simulink model "sampleModel298"  (R2021b)
settings: Solver=VariableStepAuto  StartTime=0.0  StopTime=10.0  RelTol=1e-3
libraries: simulink x11, slpidlib x2
settings Model: Creator=user  LastModifiedBy=user

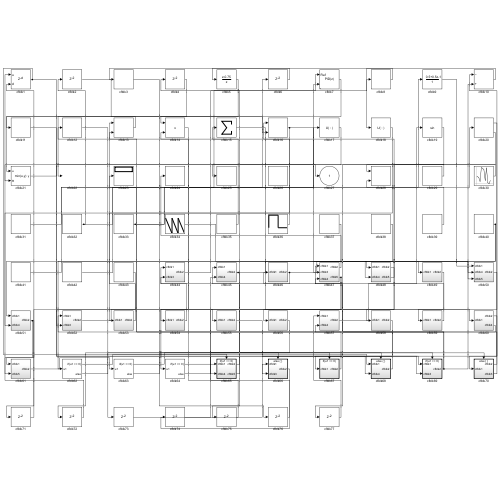
[thumbnail: Simulink's stored preview of the top-level diagram]
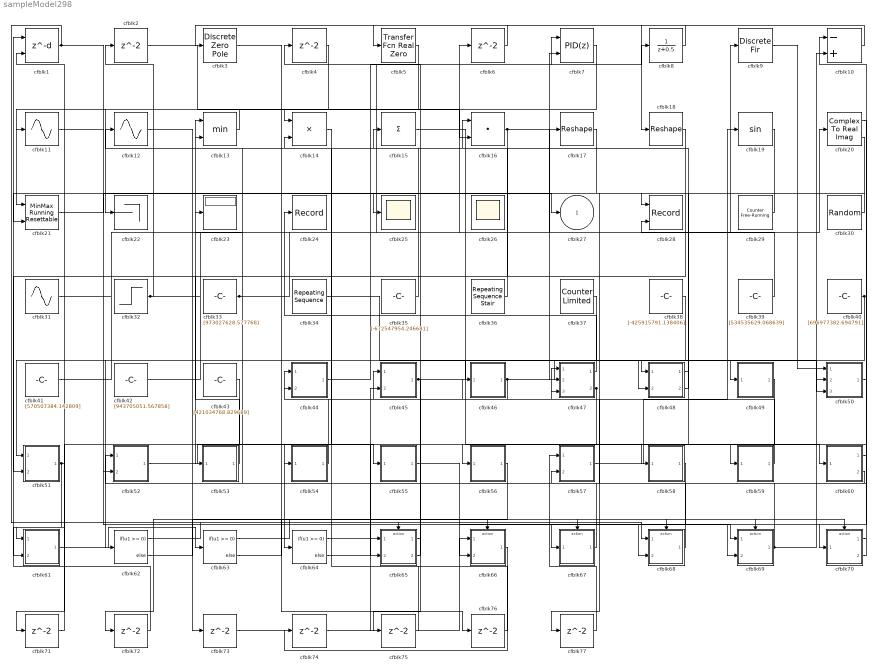
== system sampleModel298 ==
  cfblk1 : Delay  DelayLengthSource=Input port  SampleTime=1
      settings: InputPortMap=u0,p1
  cfblk10 : Sum  Inputs=-+
  cfblk11 : Sin  TimeSource=Use external signal  SampleTime=0
  cfblk12 : Sin  TimeSource=Use external signal  SampleTime=0
  cfblk13 : MinMax  Inputs=2
  cfblk14 : Product
  cfblk15 : Sum  Inputs=+
  cfblk16 : DotProduct  InputSameDT=on  OutDataTypeStr=Inherit: Inherit via internal rule
  cfblk17 : Reshape
  cfblk18 : Reshape
  cfblk19 : Trigonometry
  cfblk{2,4,6,71..77} (10 alike) : Delay  SampleTime=1
  cfblk20 : ComplexToRealImag
  cfblk21 : simulink/Math Operations/MinMax Running Resettable  Function=min  vinit=0.0
  cfblk22 : Terminator
  cfblk23 : Display
  cfblk24 : Record  FileSettingsInternal="{\"entries\":[{\"content\":{\"excelSettings\":{\"content\":{},\"type\":\"Streamout.ExcelSettings\"}},\"type\":\"Streamout.FileSettingStorage\",\"uuid\":\"f8e03bbd-3925-4cbe-a2d8-1c15d8116227\"}],\"packageUris\":[\"http://schema.mathworks.com/mf0/streamout_blocks/R2020a\"],\"version\":\"1.0\"}"  SignalsInternal="{\"entries\":[{\"content\":{\"signals\":[{\"content\":{\"blockPath\":[\"sampleModel298/cfblk24\"],\"channel\":[],\"dimensions\":[1],\"domain\":\"sampleModel298/cfblk24\",\"lineColor\":\"#a2142f\",\"plots\":[1],\"port\":1,\"sid\":[\"\"],\"signalID\":12860,\"signalName\":\"cfblk47:1\"},\"type\":\"RecordBlkView.Signal\",\"uuid\":\"11e5b281-7313-45d0-8552-5ee48f4d8115\"}]},\"type\":\"RecordBlkView.InputSignals\",\"uuid\":\"8eee72e8-d15a-4497-b3c0-09b01b3c1e58\"}],\"packageUris\":[\"http://schema.mathworks.com/mf0/streamout_blocks/R2020a\"],\"version\":\"1.0\"}"  VisualizationBindings="{\"sparklinesplugin\":{\"info\":[{\"bindingParametersList\":[],\"subplotID\":1}]}}"
  cfblk25 : Scope
  cfblk26 : Scope
      settings: Floating=on
  cfblk28 : Record  FileSettingsInternal="{\"entries\":[{\"content\":{\"excelSettings\":{\"content\":{},\"type\":\"Streamout.ExcelSettings\"}},\"type\":\"Streamout.FileSettingStorage\",\"uuid\":\"aa3ee1ba-3106-412b-81ca-2127dd02a330\"}],\"packageUris\":[\"http://schema.mathworks.com/mf0/streamout_blocks/R2020a\"],\"version\":\"1.0\"}"  Layout=[1 1]  SignalsInternal="{\"entries\":[{\"content\":{\"signals\":[{\"content\":{\"blockPath\":[\"sampleModel298/cfblk28\"],\"channel\":[],\"dimensions\":[1],\"domain\":\"sampleModel298/cfblk28\",\"lineColor\":\"#a2142f\",\"plots\":[1],\"port\":1,\"sid\":[\"\"],\"signalID\":12864,\"signalName\":\"cfblk30\"},\"type\":\"RecordBlkView.Signal\",\"uuid\":\"5ab1b331-6bbc-4e8d-9462-f5e53011d17e\"},{\"content\":{\"blockPath\":[\"sampleModel298/cfblk28\"],\"channel\":[],\"dimensions\":[1],\"domain\":\"sampleModel298/cfblk28\",\"lineColor\":\"#139fff\",\"plots\":[1],\"port\":2,\"sid\":[\"\"],\"signalID\":12868,\"signalName\":\"cfblk39\"},\"type\":\"RecordBlkView.Signal\",\"uuid\":\"ca5edff8-c0fa-4e9c-811a-b661a9ca84b8\"}]},\"type\":\"RecordBlkView.InputSignals\",\"uuid\":\"61fdf1d2-9825-4d1b-a59d-4a14db1b4992\"}],\"packageUris\":[\"http://schema.mathworks.com/mf0/streamout_blocks/R2020a\"],\"version\":\"1.0\"}"  VisualizationBindings="{\"xyplotplugin\":{\"info\":[{\"series\":[{\"bindingParametersList\":[{\"parameter\":\"X-Axis\",\"signalID\":12864,\"signalName\":\"cfblk30\"},{\"parameter\":\"Y-Axis\",\"signalID\":12868,\"signalName\":\"cfblk39\"}],\"seriesID\":55334}],\"subplotID\":1}]}}"  CompatibilityTag=XY
  cfblk29 : simulink/Sources/Counter Free-Running  NumBits=[26.000000]  tsamp=-1
  cfblk3 : DiscreteZeroPole  Poles=[0 0.5]  Gain=1
  cfblk30 : RandomNumber  Mean=[-77149.220000]  Variance=[41680.275805]  Seed=[340606104.000000]  SampleTime=0.1
  cfblk31 : Sin  Amplitude=[967904790.389444]  Bias=[-694401713.764800]  SampleTime=0
  cfblk32 : Step  Time=[28.000000]  Before=[-871235636.671696]  After=[850693744.630323]  SampleTime=0
  cfblk33 : Constant  Value=[973027628.577768]  SampleTime=1
  cfblk34 : simulink/Sources/Repeating Sequence  rep_seq_t=[0 2]  rep_seq_y=[-129325403.939381, -689316704.616454]
  cfblk35 : Constant  Value=[-672547954.246681]  SampleTime=1
  cfblk36 : simulink/Sources/Repeating Sequence Stair  OutValues=[-374108966.270243, -413875160.469731]  tsamp=-1  OutMin=[]  OutMax=[]  OutDataTypeStr=double  OutputDataTypeScalingMode=double  OutDataType=fixdt(0,8)  ConRadixGroup=Best Precision: Vector-wise  OutScaling=2^-12
  cfblk37 : simulink/Sources/Counter Limited  uplimit=[389.000000]  tsamp=-1
  cfblk38 : Constant  Value=[-425915791.138406]  SampleTime=1
  cfblk39 : Constant  Value=[534535629.068639]  SampleTime=1
  cfblk40 : Constant  Value=[696977382.694791]  SampleTime=1
  cfblk41 : Constant  Value=[570507384.142809]  SampleTime=1
  cfblk42 : Constant  Value=[943705051.567858]  SampleTime=1
  cfblk43 : Constant  Value=[421034768.829689]  SampleTime=1
  cfblk44 : Subsystem
  cfblk45 : Subsystem
  cfblk46 : Subsystem
  cfblk47 : Subsystem
  cfblk48 : Subsystem
  cfblk49 : Subsystem
  cfblk5 : simulink/Discrete/Transfer Fcn Real Zero  ZeroZ=0.75  ICPrevInput=0.0  DoSatur=off
      settings: SourceProductBaseCode=SL
  cfblk50 : Subsystem
  cfblk51 : Subsystem
  cfblk52 : Subsystem
  cfblk53 : Subsystem
  cfblk54 : Subsystem
  cfblk55 : Subsystem
  cfblk56 : Subsystem
  cfblk57 : Subsystem
  cfblk58 : Subsystem
  cfblk59 : Subsystem
  cfblk60 : Subsystem
  cfblk61 : Subsystem
  cfblk62 : If  IfExpression=u1 >= 0  SampleTime=1
  cfblk63 : If  IfExpression=u1 >= 0  SampleTime=1
  cfblk64 : If  IfExpression=u1 >= 0  SampleTime=1
  cfblk65 : Subsystem  TreatAsAtomicUnit=on
  cfblk66 : Subsystem  TreatAsAtomicUnit=on
  cfblk67 : Subsystem  TreatAsAtomicUnit=on
  cfblk68 : Subsystem  TreatAsAtomicUnit=on
  cfblk69 : Subsystem  TreatAsAtomicUnit=on
  cfblk7 : slpidlib/PID Controller (2DOF)  Controller=PID  Form=Parallel  TimeDomain=Discrete-time  UseExternalTs=off  SampleTime=1  IntegratorMethod=Forward Euler  FilterMethod=Forward Euler  ControllerParametersSource=internal  P=1  I=1  D=0  UseFilter=on  N=100  b=1  c=1  TunerSelectOption=Transfer Function Based (PID Tuner App)  InitialConditionSource=internal  InitialConditionForIntegrator=0  InitialConditionForFilter=0  DifferentiatorICPrevScaledInput=0  ExternalReset=none  TrackingMode=off  Kt=1  LimitOutput=off  SatLimitsSource=internal  UpperSaturationLimit=inf  LowerSaturationLimit=-inf  LinearizeAsGain=off  AntiWindupMode=none  Kb=1  POutMin=[]  POutMax=[]  IOutMin=[]  IOutMax=[]  DOutMin=[]  DOutMax=[]  NOutMin=[]  NOutMax=[]  bOutMin=[]  bOutMax=[]  cOutMin=[]  cOutMax=[]  SumOutMin=[]  SumOutMax=[]  SaturationOutMin=[]  SaturationOutMax=[]  PParamMin=[]  PParamMax=[]  IParamMin=[]  IParamMax=[]  DParamMin=[]  DParamMax=[]  NParamMin=[]  NParamMax=[]  bParamMin=[]  bParamMax=[]  cParamMin=[]  cParamMax=[]  KbParamMin=[]  KbParamMax=[]  KtParamMin=[]  KtParamMax=[]  KbOutMin=[]  KbOutMax=[]  KtOutMin=[]  KtOutMax=[]  IntegratorOutMin=[]  IntegratorOutMax=[]  FilterOutMin=[]  FilterOutMax=[]  SumI1OutMin=[]  SumI1OutMax=[]  SumI2OutMin=[]  SumI2OutMax=[]  SumI3OutMin=[]  SumI3OutMax=[]  SumI4OutMin=[]  SumI4OutMax=[]  SumDOutMin=[]  SumDOutMax=[]  Sum1OutMin=[]  Sum1OutMax=[]  Sum2OutMin=[]  Sum2OutMax=[]  Sum3OutMin=[]  Sum3OutMax=[]  DifferentiatorOutMin=[]  DifferentiatorOutMax=[]  FilterDiffOutCoefMin=[]  FilterDiffOutCoefMax=[]  ReciprocalOutMin=[]  ReciprocalOutMax=[]  SumDenOutMin=[]  SumDenOutMax=[]  SumNumOutMin=[]  SumNumOutMax=[]  DivideOutMin=[]  DivideOutMax=[]  UdiffTsProdOutMin=[]  UdiffTsProdOutMax=[]  NTsProdOutMin=[]  NTsProdOutMax=[]  UintegralTsProdOutMin=[]  UintegralTsProdOutMax=[]  UngainTsProdOutMin=[]  UngainTsProdOutMax=[]  IntegratorContinuousStateAttributes=''  IntegratorStateMustResolveToSignalObject=off  IntegratorRTWStateStorageClass=Auto  FilterContinuousStateAttributes=''  FilterStateMustResolveToSignalObject=off  FilterRTWStateStorageClass=Auto  ParallelPVariant=InternalParameters  IdealPVariant=Disabled  IVariant=InternalParameters  DVariant=InternalParameters  bVariant=InternalParameters  cVariant=InternalParameters  IntegratorVariant=Discrete  SatVariant=Disabled  AWVariant=Passthrough  PCopyVariant=Disabled  TRVariant=Disabled  FdbkBlocksVariant=Forward  IdealPFdbkVariant=Disabled  SatFdbkVariant=Disabled  DerivativeFilterVariant=ForwardEulerFilter  NVariant=InternalParameters  NCopyVariant=Disabled  FilterICVariant=InternalICsFilter  IntegratorICVariant=InternalICs  ExternalResetVariant=Disabled  TRSumVariant=Passthrough  SumFdbkVariant=Disabled  SumVariant=Sum_PID  TsampFilterVariant=InternalTs  TsampNgainVariant=Passthrough  TsampIntegralVariant=Passthrough  ExternalSaturationOutDataTypeStr=Inherit: Same as second input
      settings: SourceProductBaseCode=SL
  cfblk70 : Subsystem  TreatAsAtomicUnit=on
  cfblk8 : DiscreteTransferFcn  SampleTime=1
  cfblk9 : DiscreteFir  SampleTime=1
  cfblk27 : Outport
  wires:
  cfblk15/1 -> cfblk60/1(cfblk1)
  cfblk70/1(cfblk2) -> cfblk10/1
  cfblk50/1(cfblk2) -> cfblk70/1(cfblk1)
  cfblk20/1 -> cfblk59/1(cfblk1)
  cfblk31/1 -> cfblk7/1
  cfblk52/1(cfblk2) -> cfblk55/1(cfblk1)
  cfblk53/1(cfblk2) -> cfblk13/1
  cfblk9/1 -> cfblk50/1(cfblk1)
  cfblk13/1 -> cfblk22/1
  cfblk69/1(cfblk2) -> cfblk10/2, cfblk47/1(cfblk1), cfblk47/3(cfblk4)
  cfblk30/1 -> cfblk28/1
  cfblk54/1(cfblk2) -> cfblk44/1(cfblk1)
  cfblk61/1(cfblk2) -> cfblk63/1
  cfblk1/1 -> cfblk68/1(cfblk1), cfblk69/2(cfblk3)
  cfblk40/1 -> cfblk51/1(cfblk1), cfblk47/2(cfblk3)
  cfblk21/1 -> cfblk27/1
  cfblk16/1 -> cfblk53/1(cfblk1), cfblk50/3(cfblk5)
  cfblk65/1(cfblk2) -> cfblk45/1(cfblk1)
  cfblk10/1 -> cfblk18/1
  cfblk51/1(cfblk2) -> cfblk61/2(cfblk5), cfblk71/1
  cfblk4/1 -> cfblk14/1
  cfblk18/1 -> cfblk51/2(cfblk4)
  cfblk29/1 -> cfblk25/1
  cfblk41/1 -> cfblk9/1
  cfblk45/1(cfblk2) -> cfblk48/1(cfblk1), cfblk75/1
  cfblk36/1 -> cfblk16/1
  cfblk46/1(cfblk2) -> cfblk49/1(cfblk1), cfblk44/2(cfblk3)
  cfblk48/1(cfblk2) -> cfblk56/1(cfblk1)
  cfblk48/2(cfblk5) -> cfblk12/1
  cfblk60/1(cfblk2) -> cfblk67/1(cfblk1)
  cfblk35/1 -> cfblk15/1
  cfblk5/1 -> cfblk21/1
  cfblk67/1(cfblk2) -> cfblk23/1
  cfblk33/1 -> cfblk7/2, cfblk6/1
  cfblk47/1(cfblk2) -> cfblk24/1
  cfblk7/1 -> cfblk11/1
  cfblk55/1(cfblk2) -> cfblk68/2(cfblk4)
  cfblk39/1 -> cfblk28/2
  cfblk58/1(cfblk2) -> cfblk66/2(cfblk3)
  cfblk17/1 -> cfblk21/2
  cfblk32/1 -> cfblk2/1, cfblk17/1
  cfblk57/1(cfblk2) -> cfblk19/1
  cfblk44/1(cfblk2) -> cfblk8/1
  cfblk49/1(cfblk2) -> cfblk64/1
  cfblk6/1 -> cfblk5/1
  cfblk47/2(cfblk5) -> cfblk61/1(cfblk1), cfblk65/2(cfblk4)
  cfblk60/2(cfblk4) -> cfblk57/2(cfblk4)
  cfblk20/2 -> cfblk58/1(cfblk1)
  cfblk37/1 -> cfblk62/1
  cfblk38/1 -> cfblk48/2(cfblk4)
  cfblk2/1 -> cfblk16/2
  cfblk70/2(cfblk3) -> cfblk52/1(cfblk1)
  cfblk42/1 -> cfblk20/1
  cfblk68/1(cfblk2) -> cfblk13/2
  cfblk34/1 -> cfblk50/2(cfblk4)
  cfblk8/1 -> cfblk3/1
  cfblk59/1(cfblk2) -> cfblk46/1(cfblk1)
  cfblk43/1 -> cfblk52/2(cfblk3)
  cfblk65/2(cfblk5) -> cfblk4/1
  cfblk14/1 -> cfblk54/1(cfblk1)
  cfblk11/1 -> cfblk69/1(cfblk1)
  cfblk62/1 -> cfblk65/Action
  cfblk62/2 -> cfblk66/Action
  cfblk63/1 -> cfblk67/Action
  cfblk63/2 -> cfblk68/Action
  cfblk64/1 -> cfblk69/Action
  cfblk64/2 -> cfblk70/Action
  cfblk71/1 -> cfblk1/2
  cfblk56/1(cfblk2) -> cfblk72/1
  cfblk72/1 -> cfblk1/1
  cfblk12/1 -> cfblk73/1
  cfblk73/1 -> cfblk66/1(cfblk1)
  cfblk66/1(cfblk2) -> cfblk74/1
  cfblk74/1 -> cfblk45/2(cfblk4)
  cfblk75/1 -> cfblk65/1(cfblk1)
  cfblk3/1 -> cfblk76/1
  cfblk76/1 -> cfblk14/2
  cfblk19/1 -> cfblk77/1
  cfblk77/1 -> cfblk57/1(cfblk1)

== system sampleModel298/cfblk44 ==
  cfblk1 : Inport
  cfblk3 : Inport  Port=2
  cfblk2 : Outport
  wires:
  cfblk1/1 -> cfblk2/1

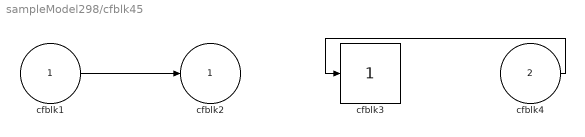
== system sampleModel298/cfblk45 ==
  cfblk1 : Inport
  cfblk4 : Inport  Port=2
  cfblk3 : simulink/Math Operations/Slider Gain  gain=1  low=0  high=2
  cfblk2 : Outport
  wires:
  cfblk1/1 -> cfblk2/1
  cfblk4/1 -> cfblk3/1

== system sampleModel298/cfblk46 ==
  cfblk1 : Inport
  cfblk3 : ComplexToMagnitudeAngle
  cfblk2 : Outport
  wires:
  cfblk3/1 -> cfblk2/1
  cfblk1/1 -> cfblk3/1

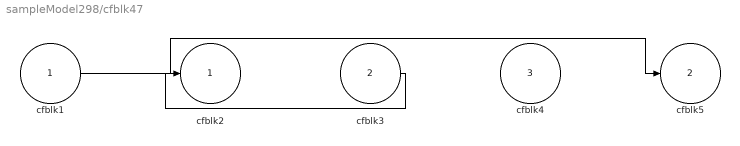
== system sampleModel298/cfblk47 ==
  cfblk1 : Inport
  cfblk3 : Inport  Port=2
  cfblk4 : Inport  Port=3
  cfblk2 : Outport
  cfblk5 : Outport  Port=2
  wires:
  cfblk1/1 -> cfblk5/1
  cfblk3/1 -> cfblk2/1

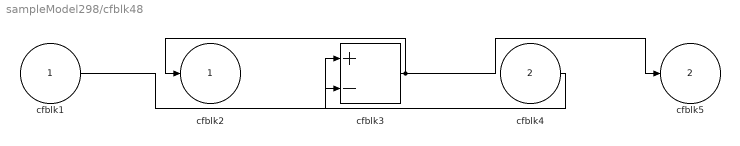
== system sampleModel298/cfblk48 ==
  cfblk1 : Inport
  cfblk4 : Inport  Port=2
  cfblk3 : Sum  Inputs=+-
  cfblk2 : Outport
  cfblk5 : Outport  Port=2
  wires:
  cfblk3/1 -> cfblk2/1, cfblk5/1
  cfblk1/1 -> cfblk3/1
  cfblk4/1 -> cfblk3/2

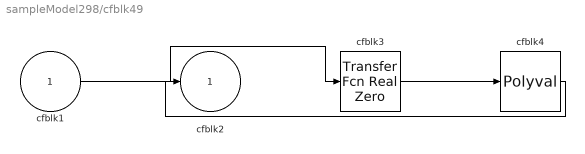
== system sampleModel298/cfblk49 ==
  cfblk1 : Inport
  cfblk3 : simulink/Discrete/Transfer Fcn Real Zero  ZeroZ=0.75  ICPrevInput=0.0  DoSatur=off
      settings: SourceProductBaseCode=SL
  cfblk4 : Polyval  Coefs=[ +2.081618890e-019, -1.441693666e-014, +4.719686976e-010, -8.536869453e-006, +1.621573104e-001, -8.087801117e+001 ]
  cfblk2 : Outport
  wires:
  cfblk3/1 -> cfblk4/1
  cfblk1/1 -> cfblk3/1
  cfblk4/1 -> cfblk2/1

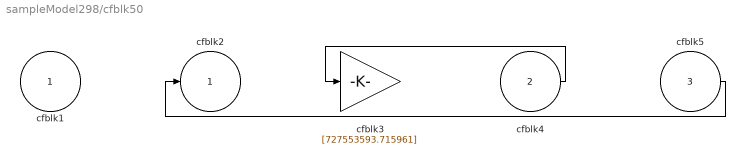
== system sampleModel298/cfblk50 ==
  cfblk1 : Inport
  cfblk4 : Inport  Port=2
  cfblk5 : Inport  Port=3
  cfblk3 : Gain  Gain=[727553593.715961]
  cfblk2 : Outport
  wires:
  cfblk4/1 -> cfblk3/1
  cfblk5/1 -> cfblk2/1

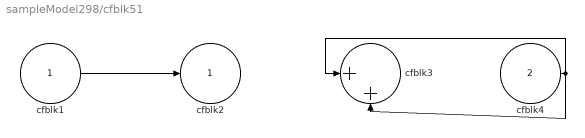
== system sampleModel298/cfblk51 ==
  cfblk1 : Inport
  cfblk4 : Inport  Port=2
  cfblk3 : Sum  Inputs=|++
  cfblk2 : Outport
  wires:
  cfblk1/1 -> cfblk2/1
  cfblk4/1 -> cfblk3/1, cfblk3/2

== system sampleModel298/cfblk52 ==
  cfblk1 : Inport
  cfblk3 : Inport  Port=2
  cfblk2 : Outport
  wires:
  cfblk3/1 -> cfblk2/1

== system sampleModel298/cfblk53 ==
  cfblk1 : Inport
  cfblk3 : DotProduct  InputSameDT=on  OutDataTypeStr=Inherit: Inherit via internal rule
  cfblk2 : Outport
  wires:
  cfblk1/1 -> cfblk3/1, cfblk3/2
  cfblk3/1 -> cfblk2/1

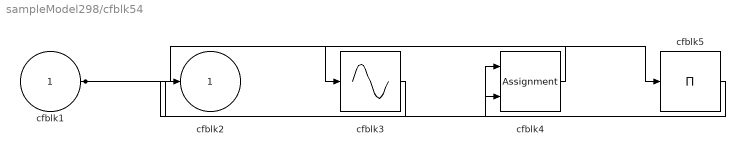
== system sampleModel298/cfblk54 ==
  cfblk1 : Inport
  cfblk3 : Sin  TimeSource=Use external signal  SampleTime=0
  cfblk4 : Assignment  DiagnosticForDimensions=Warning  IndexOptions=Index vector (dialog)  Indices=1  OutputSizes=1
  cfblk5 : Product  Inputs=*
  cfblk2 : Outport
  wires:
  cfblk1/1 -> cfblk5/1, cfblk4/2
  cfblk3/1 -> cfblk2/1
  cfblk4/1 -> cfblk3/1
  cfblk5/1 -> cfblk4/1

== system sampleModel298/cfblk55 ==
  cfblk1 : Inport
  cfblk3 : Rounding
  cfblk2 : Outport
  wires:
  cfblk1/1 -> cfblk3/1
  cfblk3/1 -> cfblk2/1

== system sampleModel298/cfblk56 ==
  cfblk1 : Inport
  cfblk3 : Polyval  Coefs=[ +2.081618890e-019, -1.441693666e-014, +4.719686976e-010, -8.536869453e-006, +1.621573104e-001, -8.087801117e+001 ]
  cfblk2 : Outport
  wires:
  cfblk1/1 -> cfblk2/1, cfblk3/1

== system sampleModel298/cfblk57 ==
  cfblk1 : Inport
  cfblk4 : Inport  Port=2
  cfblk3 : simulink/Math Operations/Slider Gain  gain=1  low=0  high=2
  cfblk2 : Outport
  wires:
  cfblk3/1 -> cfblk2/1
  cfblk1/1 -> cfblk3/1

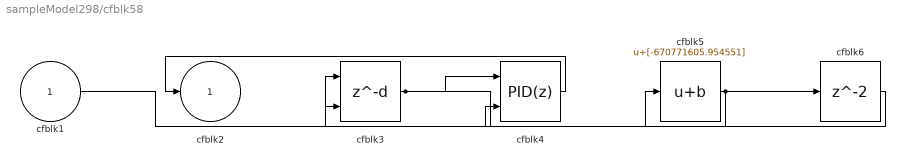
== system sampleModel298/cfblk58 ==
  cfblk1 : Inport
  cfblk3 : Delay  DelayLengthSource=Input port  SampleTime=1
      settings: InputPortMap=u0,p1
  cfblk4 : slpidlib/PID Controller (2DOF)  Controller=PID  Form=Parallel  TimeDomain=Discrete-time  UseExternalTs=off  SampleTime=1  IntegratorMethod=Forward Euler  FilterMethod=Forward Euler  ControllerParametersSource=internal  P=1  I=1  D=0  UseFilter=on  N=100  b=1  c=1  TunerSelectOption=Transfer Function Based (PID Tuner App)  InitialConditionSource=internal  InitialConditionForIntegrator=0  InitialConditionForFilter=0  DifferentiatorICPrevScaledInput=0  ExternalReset=none  TrackingMode=off  Kt=1  LimitOutput=off  SatLimitsSource=internal  UpperSaturationLimit=inf  LowerSaturationLimit=-inf  LinearizeAsGain=off  AntiWindupMode=none  Kb=1  POutMin=[]  POutMax=[]  IOutMin=[]  IOutMax=[]  DOutMin=[]  DOutMax=[]  NOutMin=[]  NOutMax=[]  bOutMin=[]  bOutMax=[]  cOutMin=[]  cOutMax=[]  SumOutMin=[]  SumOutMax=[]  SaturationOutMin=[]  SaturationOutMax=[]  PParamMin=[]  PParamMax=[]  IParamMin=[]  IParamMax=[]  DParamMin=[]  DParamMax=[]  NParamMin=[]  NParamMax=[]  bParamMin=[]  bParamMax=[]  cParamMin=[]  cParamMax=[]  KbParamMin=[]  KbParamMax=[]  KtParamMin=[]  KtParamMax=[]  KbOutMin=[]  KbOutMax=[]  KtOutMin=[]  KtOutMax=[]  IntegratorOutMin=[]  IntegratorOutMax=[]  FilterOutMin=[]  FilterOutMax=[]  SumI1OutMin=[]  SumI1OutMax=[]  SumI2OutMin=[]  SumI2OutMax=[]  SumI3OutMin=[]  SumI3OutMax=[]  SumI4OutMin=[]  SumI4OutMax=[]  SumDOutMin=[]  SumDOutMax=[]  Sum1OutMin=[]  Sum1OutMax=[]  Sum2OutMin=[]  Sum2OutMax=[]  Sum3OutMin=[]  Sum3OutMax=[]  DifferentiatorOutMin=[]  DifferentiatorOutMax=[]  FilterDiffOutCoefMin=[]  FilterDiffOutCoefMax=[]  ReciprocalOutMin=[]  ReciprocalOutMax=[]  SumDenOutMin=[]  SumDenOutMax=[]  SumNumOutMin=[]  SumNumOutMax=[]  DivideOutMin=[]  DivideOutMax=[]  UdiffTsProdOutMin=[]  UdiffTsProdOutMax=[]  NTsProdOutMin=[]  NTsProdOutMax=[]  UintegralTsProdOutMin=[]  UintegralTsProdOutMax=[]  UngainTsProdOutMin=[]  UngainTsProdOutMax=[]  IntegratorContinuousStateAttributes=''  IntegratorStateMustResolveToSignalObject=off  IntegratorRTWStateStorageClass=Auto  FilterContinuousStateAttributes=''  FilterStateMustResolveToSignalObject=off  FilterRTWStateStorageClass=Auto  ParallelPVariant=InternalParameters  IdealPVariant=Disabled  IVariant=InternalParameters  DVariant=InternalParameters  bVariant=InternalParameters  cVariant=InternalParameters  IntegratorVariant=Discrete  SatVariant=Disabled  AWVariant=Passthrough  PCopyVariant=Disabled  TRVariant=Disabled  FdbkBlocksVariant=Forward  IdealPFdbkVariant=Disabled  SatFdbkVariant=Disabled  DerivativeFilterVariant=ForwardEulerFilter  NVariant=InternalParameters  NCopyVariant=Disabled  FilterICVariant=InternalICsFilter  IntegratorICVariant=InternalICs  ExternalResetVariant=Disabled  TRSumVariant=Passthrough  SumFdbkVariant=Disabled  SumVariant=Sum_PID  TsampFilterVariant=InternalTs  TsampNgainVariant=Passthrough  TsampIntegralVariant=Passthrough  ExternalSaturationOutDataTypeStr=Inherit: Same as second input
      settings: SourceProductBaseCode=SL
  cfblk5 : Bias  Bias=[-670771605.954551]
  cfblk6 : Delay  SampleTime=1
  cfblk2 : Outport
  wires:
  cfblk4/1 -> cfblk2/1
  cfblk1/1 -> cfblk3/1
  cfblk3/1 -> cfblk5/1, cfblk4/1
  cfblk5/1 -> cfblk4/2, cfblk6/1
  cfblk6/1 -> cfblk3/2

== system sampleModel298/cfblk59 ==
  cfblk1 : Inport
  cfblk3 : simulink/Discrete/Transfer Fcn First Order  PoleZ=0.95  ICPrevOutput=0.0  DoSatur=off
  cfblk2 : Outport
  wires:
  cfblk1/1 -> cfblk3/1
  cfblk3/1 -> cfblk2/1

== system sampleModel298/cfblk60 ==
  cfblk1 : Inport
  cfblk3 : simulink/Discrete/Transfer Fcn Real Zero  ZeroZ=0.75  ICPrevInput=0.0  DoSatur=off
      settings: SourceProductBaseCode=SL
  cfblk2 : Outport
  cfblk4 : Outport  Port=2
  wires:
  cfblk1/1 -> cfblk3/1, cfblk4/1
  cfblk3/1 -> cfblk2/1

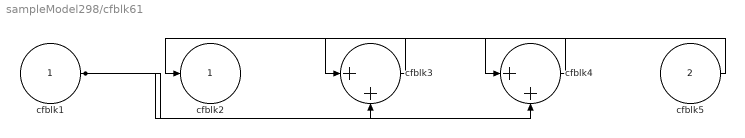
== system sampleModel298/cfblk61 ==
  cfblk1 : Inport
  cfblk5 : Inport  Port=2
  cfblk3 : Sum  Inputs=|++
  cfblk4 : Sum  Inputs=|++
  cfblk2 : Outport
  wires:
  cfblk3/1 -> cfblk2/1
  cfblk5/1 -> cfblk4/1
  cfblk1/1 -> cfblk4/2, cfblk3/2
  cfblk4/1 -> cfblk3/1

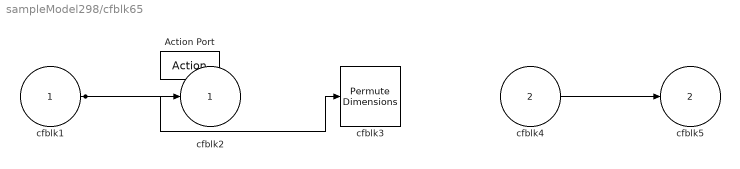
== system sampleModel298/cfblk65 ==
  cfblk1 : Inport
  cfblk4 : Inport  Port=2
  Action Port : ActionPort  ActionPortLabel=if(u1 >= 0)
  cfblk3 : PermuteDimensions
  cfblk2 : Outport
  cfblk5 : Outport  Port=2
  wires:
  cfblk4/1 -> cfblk5/1
  cfblk1/1 -> cfblk2/1, cfblk3/1

== system sampleModel298/cfblk66 ==
  cfblk1 : Inport
  cfblk3 : Inport  Port=2
  Action Port : ActionPort  ActionPortLabel=else
  cfblk2 : Outport
  wires:
  cfblk3/1 -> cfblk2/1

== system sampleModel298/cfblk67 ==
  cfblk1 : Inport
  Action Port : ActionPort  ActionPortLabel=if(u1 >= 0)
  cfblk3 : UnitDelay  SampleTime=-1  HasFrameUpgradeWarning=on
  cfblk2 : Outport
  wires:
  cfblk1/1 -> cfblk2/1, cfblk3/1

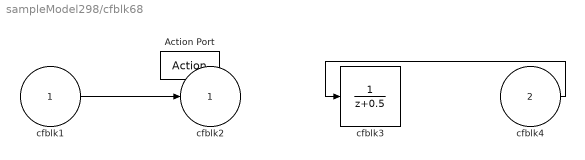
== system sampleModel298/cfblk68 ==
  cfblk1 : Inport
  cfblk4 : Inport  Port=2
  Action Port : ActionPort  ActionPortLabel=else
  cfblk3 : DiscreteTransferFcn
  cfblk2 : Outport
  wires:
  cfblk4/1 -> cfblk3/1
  cfblk1/1 -> cfblk2/1

== system sampleModel298/cfblk69 ==
  cfblk1 : Inport
  cfblk3 : Inport  Port=2
  Action Port : ActionPort  ActionPortLabel=if(u1 >= 0)
  cfblk2 : Outport
  wires:
  cfblk1/1 -> cfblk2/1

== system sampleModel298/cfblk70 ==
  cfblk1 : Inport
  Action Port : ActionPort  ActionPortLabel=else
  cfblk2 : Outport
  cfblk3 : Outport  Port=2
  wires:
  cfblk1/1 -> cfblk2/1, cfblk3/1
